simulink model "test_trajectories"  (Simulink 10.2)
settings: Solver=ode45  StartTime=0.0  StopTime=2  MaxStep=Step_Time  RelTol=1e-3  EnableMultiTasking=on
settings Model: Creator=saeed  LastModifiedBy=hosse
settings DataIOCC: LimitDataPoints=on
settings OptimizationCC: ExpressionDepthLimit=2147483647
settings DebuggingCC: SolverPrmCheckMsg=warning  StateNameClashWarn=warning  SFExecutionAtInitializationDiag=warning
settings ConfigComp: CovSFcnEnable=off

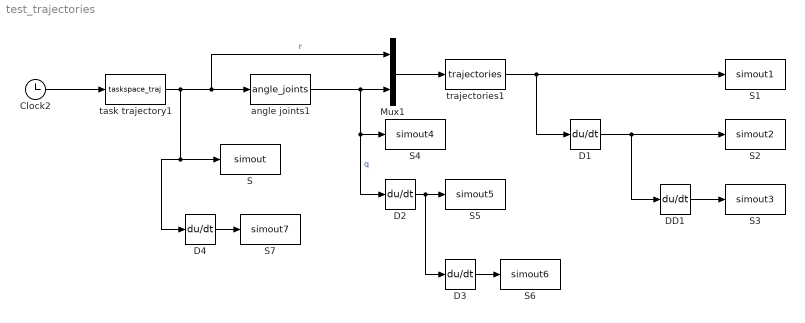
== system test_trajectories ==
  Clock2 : Clock
  D{1..4} (4 alike) : Derivative
  DD1 : Derivative
  Mux1 : Mux  Inputs=2
  S : ToWorkspace  VariableName=simout  SaveFormat=Structure With Time  SampleTime=-1
  S1 : ToWorkspace  VariableName=simout1  SaveFormat=Structure With Time  SampleTime=-1
  S2 : ToWorkspace  VariableName=simout2  SaveFormat=Structure With Time  SampleTime=-1
  S3 : ToWorkspace  VariableName=simout3  SaveFormat=Structure With Time  SampleTime=-1
  S4 : ToWorkspace  VariableName=simout4  SaveFormat=Structure With Time  SampleTime=-1
  S5 : ToWorkspace  VariableName=simout5  SaveFormat=Structure With Time  SampleTime=-1
  S6 : ToWorkspace  VariableName=simout6  SaveFormat=Structure With Time  SampleTime=-1
  S7 : ToWorkspace  VariableName=simout7  SaveFormat=Structure With Time  SampleTime=-1
  angle joints1 : MATLABFcn  MATLABFcn=angle_joints
  task trajectory1 : MATLABFcn  MATLABFcn=taskspace_traj
  trajectories1 : MATLABFcn  MATLABFcn=trajectories
  wires:
  D4/1 -> S7/1
  Clock2/1 -> task trajectory1/1
  D3/1 -> S6/1
  D2/1 -> D3/1, S5/1
  angle joints1/1 -> D2/1, S4/1, Mux1/2  "q"
  trajectories1/1 -> D1/1, S1/1
  task trajectory1/1 -> S/1, D4/1, Mux1/1, angle joints1/1  "r"
  Mux1/1 -> trajectories1/1
  DD1/1 -> S3/1
  D1/1 -> DD1/1, S2/1
